simulink model "Combined"  (R2021b)
settings: Solver=FixedStepAuto  StartTime=0.0  StopTime=inf  FixedStep=0.001  RelTol=1e-3  EnableMultiTasking=on
undefined symbols (not defined in the file): D0, D1, D10, D11, D12, D13, D2, D3, D4, D5, D6, D7, D8, D9, PTA0, PTA1, PTA2, PTB23, PTB9, PTC16, PTC17, PTC2, PTC3, PTC4, PTD0, PTD1, PTD2, PTD3
libraries: simulink x25, frdmk64flib x15
(part 1 of 2)
settings Model: ExtModeTrigDuration=5  Creator=12268  LastModifiedBy=Aaron
settings SolverCC: AlgebraicLoopSolver=TrustRegion
settings OptimizationCC: EnhancedBackFolding=on  PassReuseOutputArgsAs=Individual arguments  ZeroExternalMemoryAtStartup=off  ZeroInternalMemoryAtStartup=off  MaxStackSize=64  OptimizeBlockOrder=speed  DifferentSizesBufferReuse=on  OptimizationCustomize=off  EfficientTunableParamExpr=on
settings DebuggingCC: ParameterTunabilityLossMsg=error  SFMachineParentedDataDiag=warning
settings HardwareCC: ProdBitPerPointer=32  ProdBitPerSizeT=32  ProdBitPerPtrDiffT=32  ProdLargestAtomicInteger=Long  ProdLargestAtomicFloat=Double  ProdWordSize=32  ProdHWDeviceType=ARM Compatible->ARM Cortex
settings SFSimCC: MATLABDynamicMemAlloc=off
settings RTWCC: Description=Embedded Coder  SystemTargetFile=ert.tlc  HardwareBoard=NXP FRDM-K64F  TLCOptions="-aInlineSetEventsForThisBaseRateFcn=TLC_FALSE -aSuppressMultiTaskScheduler=TLC_FALSE  -aRateBasedStepFcn=0"  TemplateMakefile=ert_default_tmf  Toolchain=GNU Tools for ARM Embedded Processors
settings CodeAppCC: ForceParamTrailComments=on  IgnoreCustomStorageClasses=off  OperatorAnnotations=on  SimulinkDataObjDesc=on  SFDataObjDesc=on  InsertBlockDesc=on

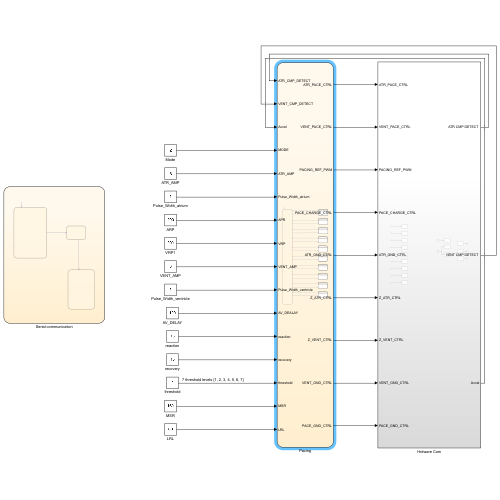
[thumbnail: Simulink's stored preview of the top-level diagram]
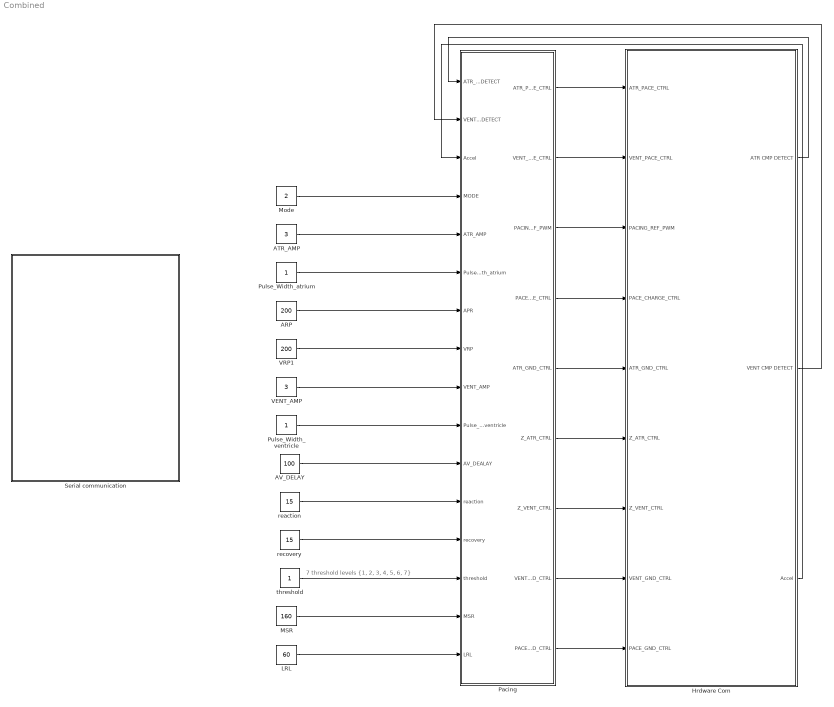
== system Combined ==
  note: 7 threshold levels {1, 2, 3, 4, 5, 6, 7}
  ARP : Constant  Value=200  OutDataTypeStr=uint16
  ATR_AMP : Constant  Value=3  OutDataTypeStr=double
  AV_DELAY : Constant  Value=100  OutDataTypeStr=uint16
  Hrdware Com : Subsystem
  LRL : Constant  Value=60
  MSR : Constant  Value=160
  Mode : Constant  Value=2  OutDataTypeStr=uint8
  Pacing : Stateflow chart  TreatAsAtomicUnit=on
      settings: PortSchema="{\"entries\":[{\"content\":{\"sides\":[{\"content\":{\"connectorIds\":[\"In1\",\"In2\",\"In3\",\"In4\",\"In5\",\"In6\",\"In8\",\"In9\",\"In16\",\"In10\",\"In11\",\"In12\",\"In13\",\"In14\",\"In15\",\"In7\"]},\"type\":\"ConnectorPlacement.EquallySpacedRectSide\",\"uuid\":\"b899f434-ac53-4776-90ad-1e47a9a70434\"},{\"content\":{\"connectorIds\":[\"Out1\",\"Out2\",\"Out3\",\"Out4\",\"Out5\",\"Out6\",\"Out7\",\"Out8\",\"Out9\"],\"side\":\"RIGHT\"},\"type\":\"ConnectorPlacement.EquallySpacedRectSide\",\"uuid\":\"a7a3dadf-3ead-4ae9-aa27-961636c111e5\"},{\"content\":{\"connectorIds\":[],\"side\":\"TOP\"},\"type\":\"ConnectorPlacement.EquallySpacedRectSide\",\"uuid\":\"97214a2f-6b07-43aa-affc-b9c6648cc812\"}]},\"type\":\"ConnectorPlacement.EquallySpacedConnector\",\"uuid\":\"1a78d035-42b2-4799-ac0c-6d5f965b7fff\"}],\"packageUris\":[\"http://schema.mathworks.com/mf0/Connector/R2020b\"],\"version\":\"1.0\"}"
  Pulse_Width_atrium : Constant  OutDataTypeStr=uint16
  Pulse_Width_ventricle : Constant  OutDataTypeStr=uint16
  Serial communication : Stateflow chart  TreatAsAtomicUnit=on
  VENT_AMP : Constant  Value=3  OutDataTypeStr=uint16
  VRP1 : Constant  Value=200  OutDataTypeStr=uint16
  reaction : Constant  Value=15  OutDataTypeStr=double
  recovery : Constant  Value=15  OutDataTypeStr=double
  threshold : Constant  OutDataTypeStr=single
  wires:
  Mode/1 -> Pacing/4(MODE)
  Pulse_Width_atrium/1 -> Pacing/6(Pulse_Width_atrium)
  ATR_AMP/1 -> Pacing/5(ATR_AMP)
  Pacing/1(ATR_PACE_CTRL) -> Hrdware Com/1(ATR_PACE_CTRL)
  Pacing/2(VENT_PACE_CTRL) -> Hrdware Com/2(VENT_PACE_CTRL)
  Pacing/3(PACING_REF_PWM) -> Hrdware Com/3(PACING_REF_PWM)
  Pacing/4(PACE_CHARGE_CTRL) -> Hrdware Com/4(PACE_CHARGE_CTRL)
  Pacing/5(ATR_GND_CTRL) -> Hrdware Com/5(ATR_GND_CTRL)
  Pacing/6(Z_ATR_CTRL) -> Hrdware Com/6("Z_ATR_CTRL ")
  Pacing/8(VENT_GND_CTRL) -> Hrdware Com/8(VENT_GND_CTRL)
  Pacing/9(PACE_GND_CTRL) -> Hrdware Com/9(PACE_GND_CTRL)
  Pacing/7(Z_VENT_CTRL) -> Hrdware Com/7("Z_VENT_CTRL ")
  ARP/1 -> Pacing/8(APR)
  Hrdware Com/1("ATR CMP DETECT ") -> Pacing/1(ATR_CMP_DETECT)
  Hrdware Com/2("VENT CMP DETECT ") -> Pacing/2(VENT_CMP_DETECT)
  VRP1/1 -> Pacing/9(VRP)
  Pulse_Width_ventricle/1 -> Pacing/10(Pulse_Width_ventricle)
  AV_DELAY/1 -> Pacing/11(AV_DEALAY)
  reaction/1 -> Pacing/12(reaction)
  threshold/1 -> Pacing/14(threshold)
  MSR/1 -> Pacing/15(MSR)
  LRL/1 -> Pacing/7(LRL)
  recovery/1 -> Pacing/13(recovery)
  Hrdware Com/3(Accel) -> Pacing/3(Accel)
  VENT_AMP/1 -> Pacing/16(VENT_AMP)

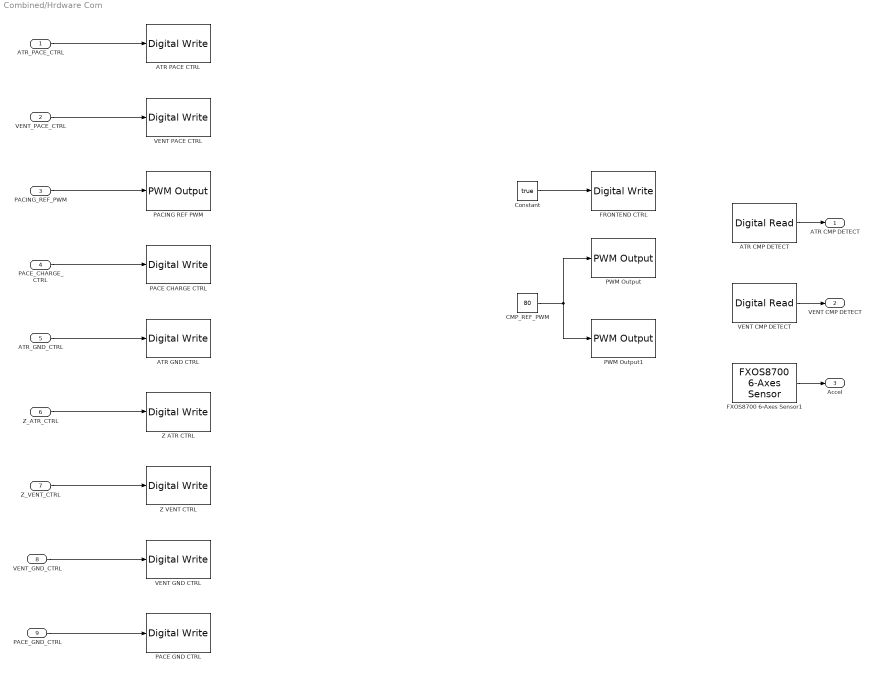
== system Combined/Hrdware Com ==
  ATR_PACE_CTRL : Inport
  VENT_PACE_CTRL : Inport  Port=2
  PACING_REF_PWM : Inport  Port=3
  PACE_CHARGE_CTRL : Inport  Port=4
  ATR_GND_CTRL : Inport  Port=5
  "Z_ATR_CTRL " : Inport  Port=6
  "Z_VENT_CTRL " : Inport  Port=7
  VENT_GND_CTRL : Inport  Port=8
  PACE_GND_CTRL : Inport  Port=9
  ATR CMP DETECT : frdmk64flib/Digital Read  Whichpin=PTC16 (D0)  SampleTime=-1
  "ATR GND CTRL " : frdmk64flib/Digital Write  Whichpin=PTD2 (D11)
  ATR PACE CTRL : frdmk64flib/Digital Write  Whichpin=PTA0 (D8)
  CMP_REF_PWM : Constant  Value=80  OutDataTypeStr=double
  Constant : Constant  Value=true  OutDataTypeStr=boolean
  FRONTEND CTRL : frdmk64flib/Digital Write  Whichpin=PTD1 (D13)
  FXOS8700 6-Axes Sensor1 : frdmk64flib/FXOS8700 6-Axes Sensor  Activesensor=Accelerometer only  ODR=800Hz  HybridODR=400Hz  Accelfullrange=-2g to +2g  SampleTime=-1
  PACE CHARGE CTRL : frdmk64flib/Digital Write  Whichpin=PTB9 (D2)
  PACE GND CTRL : frdmk64flib/Digital Write  Whichpin=PTD0 (D10)
  PACING REF PWM : frdmk64flib/PWM Output  Whichpin=PTA2 (D5)  InitialFrequency=2000  InitialDutyCycle=0
  PWM Output : frdmk64flib/PWM Output  Whichpin=PTC2 (D6)  InitialFrequency=2000  InitialDutyCycle=0
  PWM Output1 : frdmk64flib/PWM Output  Whichpin=PTA1 (D3)  InitialFrequency=2000  InitialDutyCycle=0
  VENT CMP DETECT : frdmk64flib/Digital Read  Whichpin=PTC17 (D1)  SampleTime=-1
  VENT GND CTRL : frdmk64flib/Digital Write  Whichpin=PTD3 (D12)
  VENT PACE CTRL : frdmk64flib/Digital Write  Whichpin=PTC4 (D9)
  "Z ATR CTRL " : frdmk64flib/Digital Write  Whichpin=PTB23 (D4)
  "Z VENT CTRL " : frdmk64flib/Digital Write  Whichpin=PTC3 (D7)
  "ATR CMP DETECT " : Outport  OutDataTypeStr=boolean  PortDimensions=1
  "VENT CMP DETECT " : Outport  Port=2  OutDataTypeStr=boolean  PortDimensions=1
  Accel : Outport  Port=3  OutDataTypeStr=boolean  PortDimensions=1
  wires:
  ATR_PACE_CTRL/1 -> ATR PACE CTRL/1
  VENT_PACE_CTRL/1 -> VENT PACE CTRL/1
  PACING_REF_PWM/1 -> PACING REF PWM/1
  PACE_CHARGE_CTRL/1 -> PACE CHARGE CTRL/1
  ATR_GND_CTRL/1 -> "ATR GND CTRL "/1
  "Z_ATR_CTRL "/1 -> "Z ATR CTRL "/1
  "Z_VENT_CTRL "/1 -> "Z VENT CTRL "/1
  VENT_GND_CTRL/1 -> VENT GND CTRL/1
  PACE_GND_CTRL/1 -> PACE GND CTRL/1
  Constant/1 -> FRONTEND CTRL/1
  ATR CMP DETECT/1 -> "ATR CMP DETECT "/1
  CMP_REF_PWM/1 -> PWM Output/1, PWM Output1/1
  VENT CMP DETECT/1 -> "VENT CMP DETECT "/1
  FXOS8700 6-Axes Sensor1/1 -> Accel/1

== system Combined/Pacing/AAI ==
  ATR_AMP : Inport
  Pulse_Width_atrium : Inport  Port=2
  LRL : Inport  Port=3
  APR : Inport  Port=4
  ATR_CMP_DETECT : Inport  Port=5
  Action Port : ActionPort
      settings: CopyFcn=Stateflow.SLINSF.SimulinkMan.removeBlockPreDeleteFcn  PreDeleteFcn=Stateflow.SLINSF.SimulinkMan.unsafePredeleteFcn
  "BPM to msec/B " : Subsystem
  Chart1 : Stateflow chart  TreatAsAtomicUnit=on
  ATR_PACE_CTRL : Outport
  VENT_PACE_CTRL : Outport  Port=2
  PACING_REF_PWM : Outport  Port=3
  PACE_CHARGE_CTRL : Outport  Port=4
  ATR_GND_CTRL : Outport  Port=5
  Z_ATR_CTRL : Outport  Port=6
  Z_VENT_CTRL : Outport  Port=7
  VENT_GND_CTRL : Outport  Port=8
  PACE_GND_CTRL : Outport  Port=9
  wires:
  Chart1/9(PACE_GND_CTRL) -> PACE_GND_CTRL/1
  Chart1/2(VENT_PACE_CTRL) -> VENT_PACE_CTRL/1
  Chart1/4(PACE_CHARGE_CTRL) -> PACE_CHARGE_CTRL/1
  Chart1/8(VENT_GND_CTRL) -> VENT_GND_CTRL/1
  Chart1/5(ATR_GND_CTRL) -> ATR_GND_CTRL/1
  Chart1/3(PACING_REF_PWM) -> PACING_REF_PWM/1
  Chart1/7(Z_VENT_CTRL) -> Z_VENT_CTRL/1
  Chart1/6(Z_ATR_CTRL) -> Z_ATR_CTRL/1
  Chart1/1(ATR_PACE_CTRL) -> ATR_PACE_CTRL/1
  ATR_AMP/1 -> Chart1/3(Amplitude)
  LRL/1 -> "BPM to msec/B "/1(LRL)
  Pulse_Width_atrium/1 -> Chart1/4(PULSE_WIDTH)
  APR/1 -> Chart1/2(ARP)
  "BPM to msec/B "/1(Out1) -> Chart1/5(LRL)
  ATR_CMP_DETECT/1 -> Chart1/1(SENSED)

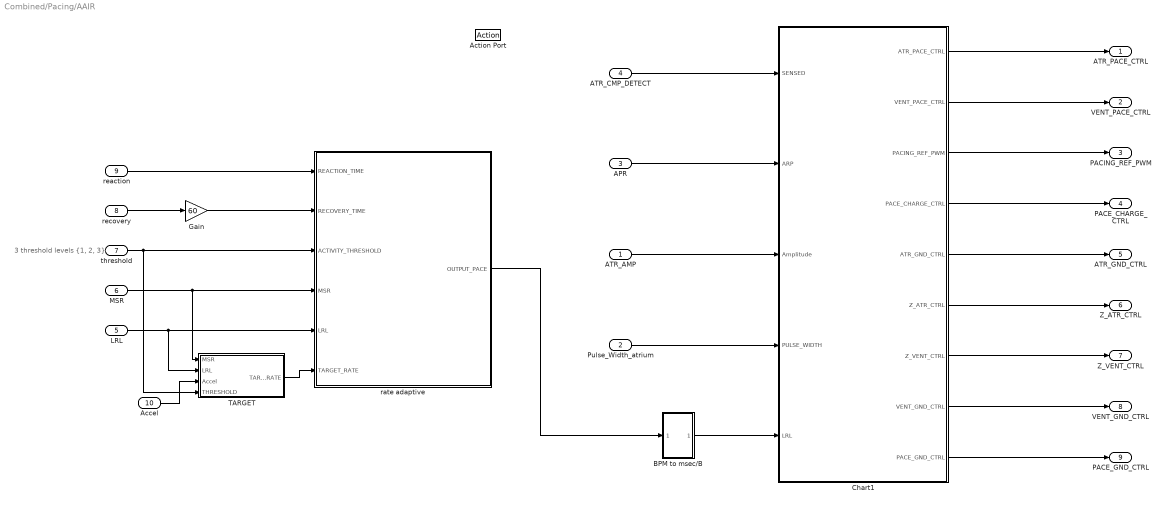
== system Combined/Pacing/AAIR ==
  note: 3 threshold levels {1, 2, 3}
  ATR_AMP : Inport
  Pulse_Width_atrium : Inport  Port=2
  APR : Inport  Port=3
  ATR_CMP_DETECT : Inport  Port=4
  LRL : Inport  Port=5
  MSR : Inport  Port=6
  threshold : Inport  Port=7
  recovery : Inport  Port=8
  reaction : Inport  Port=9
  Accel : Inport  Port=10
  Action Port : ActionPort
      settings: CopyFcn=Stateflow.SLINSF.SimulinkMan.removeBlockPreDeleteFcn  PreDeleteFcn=Stateflow.SLINSF.SimulinkMan.unsafePredeleteFcn
  "BPM to msec/B " : Subsystem
  Chart1 : Stateflow chart  TreatAsAtomicUnit=on
  Gain : Gain  Gain=60
  TARGET : Subsystem
  rate adaptive : Stateflow chart  TreatAsAtomicUnit=on
      settings: PortSchema="{\"entries\":[{\"content\":{\"sides\":[{\"content\":{\"connectorIds\":[\"In3\",\"In4\",\"In5\",\"In1\",\"In2\",\"In6\"]},\"type\":\"ConnectorPlacement.EquallySpacedRectSide\",\"uuid\":\"d3aa46b7-da68-4733-bd03-102d604fce17\"},{\"content\":{\"connectorIds\":[\"Out1\"],\"side\":\"RIGHT\"},\"type\":\"ConnectorPlacement.EquallySpacedRectSide\",\"uuid\":\"afbb636e-6b76-41fa-bb75-ca0d3f63044e\"},{\"content\":{\"connectorIds\":[],\"side\":\"TOP\"},\"type\":\"ConnectorPlacement.EquallySpacedRectSide\",\"uuid\":\"40571637-2e0f-45fd-89f0-6c332ecbd683\"}]},\"type\":\"ConnectorPlacement.EquallySpacedConnector\",\"uuid\":\"5e4e3dcb-fc0d-40cc-8fd4-4ca115cadd01\"}],\"packageUris\":[\"http://schema.mathworks.com/mf0/Connector/R2020b\"],\"version\":\"1.0\"}"
  ATR_PACE_CTRL : Outport
  VENT_PACE_CTRL : Outport  Port=2
  PACING_REF_PWM : Outport  Port=3
  PACE_CHARGE_CTRL : Outport  Port=4
  ATR_GND_CTRL : Outport  Port=5
  Z_ATR_CTRL : Outport  Port=6
  Z_VENT_CTRL : Outport  Port=7
  VENT_GND_CTRL : Outport  Port=8
  PACE_GND_CTRL : Outport  Port=9
  wires:
  recovery/1 -> Gain/1
  threshold/1 -> TARGET/4(THRESHOLD), rate adaptive/5(ACTIVITY_THRESHOLD)
  LRL/1 -> rate adaptive/2(LRL), TARGET/2(LRL)
  reaction/1 -> rate adaptive/3(REACTION_TIME)
  MSR/1 -> TARGET/1(MSR), rate adaptive/1(MSR)
  TARGET/1(TARGET_RATE) -> rate adaptive/6(TARGET_RATE)
  Gain/1 -> rate adaptive/4(RECOVERY_TIME)
  Chart1/9(PACE_GND_CTRL) -> PACE_GND_CTRL/1
  Chart1/6(Z_ATR_CTRL) -> Z_ATR_CTRL/1
  Chart1/7(Z_VENT_CTRL) -> Z_VENT_CTRL/1
  Chart1/8(VENT_GND_CTRL) -> VENT_GND_CTRL/1
  ATR_CMP_DETECT/1 -> Chart1/1(SENSED)
  Chart1/2(VENT_PACE_CTRL) -> VENT_PACE_CTRL/1
  Chart1/3(PACING_REF_PWM) -> PACING_REF_PWM/1
  Chart1/1(ATR_PACE_CTRL) -> ATR_PACE_CTRL/1
  APR/1 -> Chart1/2(ARP)
  Chart1/5(ATR_GND_CTRL) -> ATR_GND_CTRL/1
  Pulse_Width_atrium/1 -> Chart1/4(PULSE_WIDTH)
  Chart1/4(PACE_CHARGE_CTRL) -> PACE_CHARGE_CTRL/1
  "BPM to msec/B "/1(Out1) -> Chart1/5(LRL)
  rate adaptive/1(OUTPUT_PACE) -> "BPM to msec/B "/1(LRL)
  ATR_AMP/1 -> Chart1/3(Amplitude)
  Accel/1 -> TARGET/3(Accel)

== system Combined/Pacing/AOO ==
  ATR_AMP : Inport
  Pulse_Width_atrium : Inport  Port=2
  LRL : Inport  Port=3
  Action Port : ActionPort
      settings: CopyFcn=Stateflow.SLINSF.SimulinkMan.removeBlockPreDeleteFcn  PreDeleteFcn=Stateflow.SLINSF.SimulinkMan.unsafePredeleteFcn
  "BPM to msec/B " : Subsystem
  Chart : Stateflow chart  TreatAsAtomicUnit=on
  ATR_PACE_CTRL : Outport
  VENT_PACE_CTRL : Outport  Port=2
  PACING_REF_PWM : Outport  Port=3
  PACE_CHARGE_CTRL : Outport  Port=4
  ATR_GND_CTRL : Outport  Port=5
  Z_ATR_CTRL : Outport  Port=6
  Z_VENT_CTRL : Outport  Port=7
  VENT_GND_CTRL : Outport  Port=8
  PACE_GND_CTRL : Outport  Port=9
  wires:
  Chart/6(Z_ATR_CTRL) -> Z_ATR_CTRL/1
  Chart/8(VENT_GND_CTRL) -> VENT_GND_CTRL/1
  Chart/4(PACE_CHARGE_CTRL) -> PACE_CHARGE_CTRL/1
  Chart/9(PACE_GND_CTRL) -> PACE_GND_CTRL/1
  Chart/3(PACING_REF_PWM) -> PACING_REF_PWM/1
  Chart/1(ATR_PACE_CTRL) -> ATR_PACE_CTRL/1
  Chart/7(Z_VENT_CTRL) -> Z_VENT_CTRL/1
  Chart/5(ATR_GND_CTRL) -> ATR_GND_CTRL/1
  Chart/2(VENT_PACE_CTRL) -> VENT_PACE_CTRL/1
  ATR_AMP/1 -> Chart/1(Amplitude)
  Pulse_Width_atrium/1 -> Chart/2(PULSE_WIDTH)
  "BPM to msec/B "/1(Out1) -> Chart/3(LRL)
  LRL/1 -> "BPM to msec/B "/1(LRL)

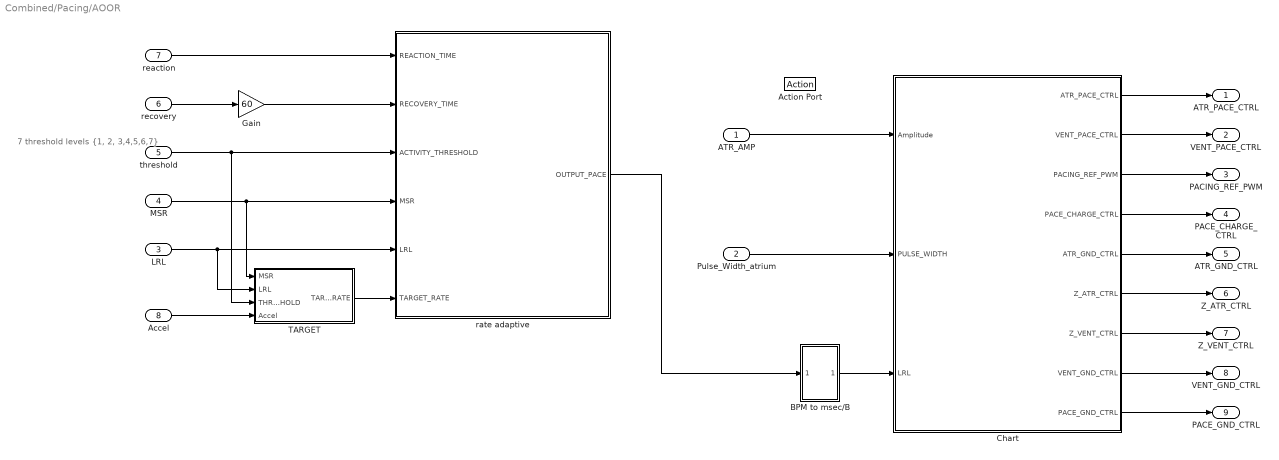
== system Combined/Pacing/AOOR ==
  note: 7 threshold levels {1, 2, 3,4,5,6,7}
  ATR_AMP : Inport
  Pulse_Width_atrium : Inport  Port=2
  LRL : Inport  Port=3
  MSR : Inport  Port=4
  threshold : Inport  Port=5
  recovery : Inport  Port=6
  reaction : Inport  Port=7
  Accel : Inport  Port=8
  Action Port : ActionPort
      settings: CopyFcn=Stateflow.SLINSF.SimulinkMan.removeBlockPreDeleteFcn  PreDeleteFcn=Stateflow.SLINSF.SimulinkMan.unsafePredeleteFcn
  "BPM to msec/B " : Subsystem
  Chart : Stateflow chart  TreatAsAtomicUnit=on
  Gain : Gain  Gain=60
  TARGET : Subsystem
  rate adaptive : Stateflow chart  TreatAsAtomicUnit=on
      settings: PortSchema="{\"entries\":[{\"content\":{\"sides\":[{\"content\":{\"connectorIds\":[\"In3\",\"In4\",\"In5\",\"In1\",\"In2\",\"In6\"]},\"type\":\"ConnectorPlacement.EquallySpacedRectSide\",\"uuid\":\"d3aa46b7-da68-4733-bd03-102d604fce17\"},{\"content\":{\"connectorIds\":[\"Out1\"],\"side\":\"RIGHT\"},\"type\":\"ConnectorPlacement.EquallySpacedRectSide\",\"uuid\":\"afbb636e-6b76-41fa-bb75-ca0d3f63044e\"},{\"content\":{\"connectorIds\":[],\"side\":\"TOP\"},\"type\":\"ConnectorPlacement.EquallySpacedRectSide\",\"uuid\":\"40571637-2e0f-45fd-89f0-6c332ecbd683\"}]},\"type\":\"ConnectorPlacement.EquallySpacedConnector\",\"uuid\":\"5e4e3dcb-fc0d-40cc-8fd4-4ca115cadd01\"}],\"packageUris\":[\"http://schema.mathworks.com/mf0/Connector/R2020b\"],\"version\":\"1.0\"}"
  ATR_PACE_CTRL : Outport
  VENT_PACE_CTRL : Outport  Port=2
  PACING_REF_PWM : Outport  Port=3
  PACE_CHARGE_CTRL : Outport  Port=4
  ATR_GND_CTRL : Outport  Port=5
  Z_ATR_CTRL : Outport  Port=6
  Z_VENT_CTRL : Outport  Port=7
  VENT_GND_CTRL : Outport  Port=8
  PACE_GND_CTRL : Outport  Port=9
  wires:
  Chart/9(PACE_GND_CTRL) -> PACE_GND_CTRL/1
  Chart/2(VENT_PACE_CTRL) -> VENT_PACE_CTRL/1
  Chart/4(PACE_CHARGE_CTRL) -> PACE_CHARGE_CTRL/1
  Chart/8(VENT_GND_CTRL) -> VENT_GND_CTRL/1
  Chart/5(ATR_GND_CTRL) -> ATR_GND_CTRL/1
  Chart/3(PACING_REF_PWM) -> PACING_REF_PWM/1
  Chart/7(Z_VENT_CTRL) -> Z_VENT_CTRL/1
  Chart/6(Z_ATR_CTRL) -> Z_ATR_CTRL/1
  Chart/1(ATR_PACE_CTRL) -> ATR_PACE_CTRL/1
  ATR_AMP/1 -> Chart/1(Amplitude)
  Pulse_Width_atrium/1 -> Chart/2(PULSE_WIDTH)
  Gain/1 -> rate adaptive/4(RECOVERY_TIME)
  "BPM to msec/B "/1(Out1) -> Chart/3(LRL)
  rate adaptive/1(OUTPUT_PACE) -> "BPM to msec/B "/1(In1)
  reaction/1 -> rate adaptive/3(REACTION_TIME)
  recovery/1 -> Gain/1
  threshold/1 -> TARGET/3(THRESHOLD), rate adaptive/5(ACTIVITY_THRESHOLD)
  MSR/1 -> TARGET/1(MSR), rate adaptive/1(MSR)
  TARGET/1(TARGET_RATE) -> rate adaptive/6(TARGET_RATE)
  LRL/1 -> rate adaptive/2(LRL), TARGET/2(LRL)
  Accel/1 -> TARGET/4(Accel)

== system Combined/Pacing/DOO ==
  VENT_AMP : Inport
  Pulse_Width_atrium : Inport  Port=2
  LRL : Inport  Port=3
  Pulse_Width_ventricle : Inport  Port=4
  AV_DEALAY : Inport  Port=5
  ATR_AMP : Inport  Port=6
  Action Port : ActionPort
      settings: CopyFcn=Stateflow.SLINSF.SimulinkMan.removeBlockPreDeleteFcn  PreDeleteFcn=Stateflow.SLINSF.SimulinkMan.unsafePredeleteFcn
  "BPM to msec/B " : Subsystem
  Chart : Stateflow chart  TreatAsAtomicUnit=on
      settings: PortSchema="{\"entries\":[{\"content\":{\"sides\":[{\"content\":{\"connectorIds\":[\"In1\",\"In6\",\"In5\",\"In2\",\"In3\",\"In4\"]},\"type\":\"ConnectorPlacement.EquallySpacedRectSide\",\"uuid\":\"72970874-2a7f-4f54-9c96-49c3612305c0\"},{\"content\":{\"connectorIds\":[\"Out1\",\"Out2\",\"Out3\",\"Out4\",\"Out5\",\"Out6\",\"Out7\",\"Out8\",\"Out9\"],\"side\":\"RIGHT\"},\"type\":\"ConnectorPlacement.EquallySpacedRectSide\",\"uuid\":\"785d6d73-c00d-4bb6-bac4-9062a7713100\"},{\"content\":{\"connectorIds\":[],\"side\":\"TOP\"},\"type\":\"ConnectorPlacement.EquallySpacedRectSide\",\"uuid\":\"f7c58201-4adc-48cf-bf7a-118db90373b1\"}]},\"type\":\"ConnectorPlacement.EquallySpacedConnector\",\"uuid\":\"33960bc4-ecd9-4e8c-b37b-5f7b6e376475\"}],\"packageUris\":[\"http://schema.mathworks.com/mf0/Connector/R2020b\"],\"version\":\"1.0\"}"
  ATR_PACE_CTRL : Outport
  VENT_PACE_CTRL : Outport  Port=2
  PACING_REF_PWM : Outport  Port=3
  PACE_CHARGE_CTRL : Outport  Port=4
  ATR_GND_CTRL : Outport  Port=5
  Z_ATR_CTRL : Outport  Port=6
  Z_VENT_CTRL : Outport  Port=7
  VENT_GND_CTRL : Outport  Port=8
  PACE_GND_CTRL : Outport  Port=9
  wires:
  Chart/9(PACE_GND_CTRL) -> PACE_GND_CTRL/1
  AV_DEALAY/1 -> Chart/5(AV_DELAY)
  "BPM to msec/B "/1(Out1) -> Chart/4(INTERVAL)
  Chart/3(PACING_REF_PWM) -> PACING_REF_PWM/1
  Pulse_Width_atrium/1 -> Chart/3(ATR_PULSE_WIDTH)
  Chart/8(VENT_GND_CTRL) -> VENT_GND_CTRL/1
  VENT_AMP/1 -> Chart/1(V_Amplitude)
  LRL/1 -> "BPM to msec/B "/1(In1)
  Chart/5(ATR_GND_CTRL) -> ATR_GND_CTRL/1
  Chart/4(PACE_CHARGE_CTRL) -> PACE_CHARGE_CTRL/1
  Chart/2(VENT_PACE_CTRL) -> VENT_PACE_CTRL/1
  Pulse_Width_ventricle/1 -> Chart/2(VENT_PULSE_WIDTH)
  Chart/1(ATR_PACE_CTRL) -> ATR_PACE_CTRL/1
  Chart/6(Z_ATR_CTRL) -> Z_ATR_CTRL/1
  Chart/7(Z_VENT_CTRL) -> Z_VENT_CTRL/1
  ATR_AMP/1 -> Chart/6(A_Amplitude)

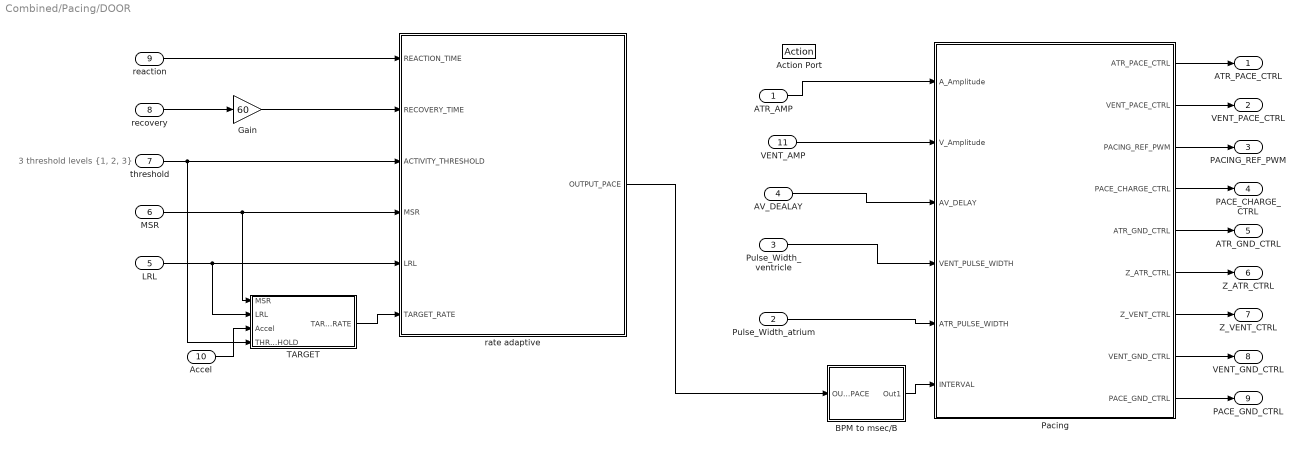
== system Combined/Pacing/DOOR ==
  note: 3 threshold levels {1, 2, 3}
  ATR_AMP : Inport
  Pulse_Width_atrium : Inport  Port=2
  Pulse_Width_ventricle : Inport  Port=3
  AV_DEALAY : Inport  Port=4
  LRL : Inport  Port=5
  MSR : Inport  Port=6
  threshold : Inport  Port=7
  recovery : Inport  Port=8
  reaction : Inport  Port=9
  Accel : Inport  Port=10
  VENT_AMP : Inport  Port=11
  Action Port : ActionPort
      settings: CopyFcn=Stateflow.SLINSF.SimulinkMan.removeBlockPreDeleteFcn  PreDeleteFcn=Stateflow.SLINSF.SimulinkMan.unsafePredeleteFcn
  "BPM to msec/B " : Subsystem
  Gain : Gain  Gain=60
  Pacing : Stateflow chart  TreatAsAtomicUnit=on
      settings: PortSchema="{\"entries\":[{\"content\":{\"sides\":[{\"content\":{\"connectorIds\":[\"In1\",\"In6\",\"In5\",\"In2\",\"In3\",\"In4\"]},\"type\":\"ConnectorPlacement.EquallySpacedRectSide\",\"uuid\":\"72970874-2a7f-4f54-9c96-49c3612305c0\"},{\"content\":{\"connectorIds\":[\"Out1\",\"Out2\",\"Out3\",\"Out4\",\"Out5\",\"Out6\",\"Out7\",\"Out8\",\"Out9\"],\"side\":\"RIGHT\"},\"type\":\"ConnectorPlacement.EquallySpacedRectSide\",\"uuid\":\"785d6d73-c00d-4bb6-bac4-9062a7713100\"},{\"content\":{\"connectorIds\":[],\"side\":\"TOP\"},\"type\":\"ConnectorPlacement.EquallySpacedRectSide\",\"uuid\":\"f7c58201-4adc-48cf-bf7a-118db90373b1\"}]},\"type\":\"ConnectorPlacement.EquallySpacedConnector\",\"uuid\":\"33960bc4-ecd9-4e8c-b37b-5f7b6e376475\"}],\"packageUris\":[\"http://schema.mathworks.com/mf0/Connector/R2020b\"],\"version\":\"1.0\"}"
  TARGET : Subsystem
  rate adaptive : Stateflow chart  TreatAsAtomicUnit=on
      settings: PortSchema="{\"entries\":[{\"content\":{\"sides\":[{\"content\":{\"connectorIds\":[\"In3\",\"In4\",\"In5\",\"In1\",\"In2\",\"In6\"]},\"type\":\"ConnectorPlacement.EquallySpacedRectSide\",\"uuid\":\"d3aa46b7-da68-4733-bd03-102d604fce17\"},{\"content\":{\"connectorIds\":[\"Out1\"],\"side\":\"RIGHT\"},\"type\":\"ConnectorPlacement.EquallySpacedRectSide\",\"uuid\":\"afbb636e-6b76-41fa-bb75-ca0d3f63044e\"},{\"content\":{\"connectorIds\":[],\"side\":\"TOP\"},\"type\":\"ConnectorPlacement.EquallySpacedRectSide\",\"uuid\":\"40571637-2e0f-45fd-89f0-6c332ecbd683\"}]},\"type\":\"ConnectorPlacement.EquallySpacedConnector\",\"uuid\":\"5e4e3dcb-fc0d-40cc-8fd4-4ca115cadd01\"}],\"packageUris\":[\"http://schema.mathworks.com/mf0/Connector/R2020b\"],\"version\":\"1.0\"}"
  ATR_PACE_CTRL : Outport
  VENT_PACE_CTRL : Outport  Port=2
  PACING_REF_PWM : Outport  Port=3
  PACE_CHARGE_CTRL : Outport  Port=4
  ATR_GND_CTRL : Outport  Port=5
  Z_ATR_CTRL : Outport  Port=6
  Z_VENT_CTRL : Outport  Port=7
  VENT_GND_CTRL : Outport  Port=8
  PACE_GND_CTRL : Outport  Port=9
  wires:
  Pulse_Width_atrium/1 -> Pacing/3(ATR_PULSE_WIDTH)
  Pacing/6(Z_ATR_CTRL) -> Z_ATR_CTRL/1
  Pacing/5(ATR_GND_CTRL) -> ATR_GND_CTRL/1
  rate adaptive/1(OUTPUT_PACE) -> "BPM to msec/B "/1(OUTPUT_PACE)
  Pacing/7(Z_VENT_CTRL) -> Z_VENT_CTRL/1
  AV_DEALAY/1 -> Pacing/5(AV_DELAY)
  "BPM to msec/B "/1(Out1) -> Pacing/4(INTERVAL)
  ATR_AMP/1 -> Pacing/1(A_Amplitude)
  Pacing/9(PACE_GND_CTRL) -> PACE_GND_CTRL/1
  Pacing/3(PACING_REF_PWM) -> PACING_REF_PWM/1
  Pacing/8(VENT_GND_CTRL) -> VENT_GND_CTRL/1
  Pacing/1(ATR_PACE_CTRL) -> ATR_PACE_CTRL/1
  Pacing/4(PACE_CHARGE_CTRL) -> PACE_CHARGE_CTRL/1
  Pulse_Width_ventricle/1 -> Pacing/2(VENT_PULSE_WIDTH)
  Pacing/2(VENT_PACE_CTRL) -> VENT_PACE_CTRL/1
  LRL/1 -> rate adaptive/2(LRL), TARGET/2(LRL)
  threshold/1 -> TARGET/4(THRESHOLD), rate adaptive/5(ACTIVITY_THRESHOLD)
  recovery/1 -> Gain/1
  MSR/1 -> TARGET/1(MSR), rate adaptive/1(MSR)
  reaction/1 -> rate adaptive/3(REACTION_TIME)
  Gain/1 -> rate adaptive/4(RECOVERY_TIME)
  TARGET/1(TARGET_RATE) -> rate adaptive/6(TARGET_RATE)
  Accel/1 -> TARGET/3(Accel)
  VENT_AMP/1 -> Pacing/6(V_Amplitude)

== system Combined/Pacing/VOO ==
  VENT_AMP : Inport
  Pulse_Width_ventricle : Inport  Port=2
  LRL : Inport  Port=3
  Action Port : ActionPort
      settings: CopyFcn=Stateflow.SLINSF.SimulinkMan.removeBlockPreDeleteFcn  PreDeleteFcn=Stateflow.SLINSF.SimulinkMan.unsafePredeleteFcn
  "BPM to msec/B " : Subsystem
  Chart : Stateflow chart  TreatAsAtomicUnit=on
  ATR_PACE_CTRL : Outport
  VENT_PACE_CTRL : Outport  Port=2
  PACING_REF_PWM : Outport  Port=3
  PACE_CHARGE_CTRL : Outport  Port=4
  ATR_GND_CTRL : Outport  Port=5
  Z_ATR_CTRL : Outport  Port=6
  Z_VENT_CTRL : Outport  Port=7
  VENT_GND_CTRL : Outport  Port=8
  PACE_GND_CTRL : Outport  Port=9
  wires:
  Chart/9(PACE_GND_CTRL) -> PACE_GND_CTRL/1
  Chart/2(VENT_PACE_CTRL) -> VENT_PACE_CTRL/1
  Chart/4(PACE_CHARGE_CTRL) -> PACE_CHARGE_CTRL/1
  Chart/8(VENT_GND_CTRL) -> VENT_GND_CTRL/1
  Chart/5(ATR_GND_CTRL) -> ATR_GND_CTRL/1
  Chart/3(PACING_REF_PWM) -> PACING_REF_PWM/1
  Chart/7(Z_VENT_CTRL) -> Z_VENT_CTRL/1
  Chart/6(Z_ATR_CTRL) -> Z_ATR_CTRL/1
  Chart/1(ATR_PACE_CTRL) -> ATR_PACE_CTRL/1
  VENT_AMP/1 -> Chart/1(Amplitude)
  Pulse_Width_ventricle/1 -> Chart/2(PULSE_WIDTH)
  "BPM to msec/B "/1(Out1) -> Chart/3(LRL)
  LRL/1 -> "BPM to msec/B "/1(LRL)

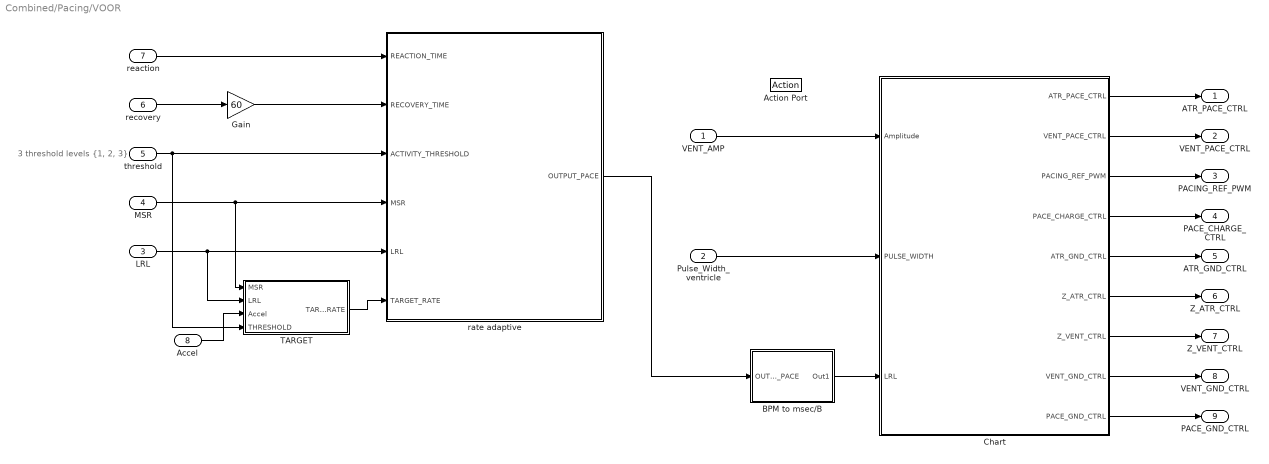
== system Combined/Pacing/VOOR ==
  note: 3 threshold levels {1, 2, 3}
  VENT_AMP : Inport
  Pulse_Width_ventricle : Inport  Port=2
  LRL : Inport  Port=3
  MSR : Inport  Port=4
  threshold : Inport  Port=5
  recovery : Inport  Port=6
  reaction : Inport  Port=7
  Accel : Inport  Port=8
  Action Port : ActionPort
      settings: CopyFcn=Stateflow.SLINSF.SimulinkMan.removeBlockPreDeleteFcn  PreDeleteFcn=Stateflow.SLINSF.SimulinkMan.unsafePredeleteFcn
  "BPM to msec/B " : Subsystem
  Chart : Stateflow chart  TreatAsAtomicUnit=on
  Gain : Gain  Gain=60
  TARGET : Subsystem
  rate adaptive : Stateflow chart  TreatAsAtomicUnit=on
      settings: PortSchema="{\"entries\":[{\"content\":{\"sides\":[{\"content\":{\"connectorIds\":[\"In3\",\"In4\",\"In5\",\"In1\",\"In2\",\"In6\"]},\"type\":\"ConnectorPlacement.EquallySpacedRectSide\",\"uuid\":\"d3aa46b7-da68-4733-bd03-102d604fce17\"},{\"content\":{\"connectorIds\":[\"Out1\"],\"side\":\"RIGHT\"},\"type\":\"ConnectorPlacement.EquallySpacedRectSide\",\"uuid\":\"afbb636e-6b76-41fa-bb75-ca0d3f63044e\"},{\"content\":{\"connectorIds\":[],\"side\":\"TOP\"},\"type\":\"ConnectorPlacement.EquallySpacedRectSide\",\"uuid\":\"40571637-2e0f-45fd-89f0-6c332ecbd683\"}]},\"type\":\"ConnectorPlacement.EquallySpacedConnector\",\"uuid\":\"5e4e3dcb-fc0d-40cc-8fd4-4ca115cadd01\"}],\"packageUris\":[\"http://schema.mathworks.com/mf0/Connector/R2020b\"],\"version\":\"1.0\"}"
  ATR_PACE_CTRL : Outport
  VENT_PACE_CTRL : Outport  Port=2
  PACING_REF_PWM : Outport  Port=3
  PACE_CHARGE_CTRL : Outport  Port=4
  ATR_GND_CTRL : Outport  Port=5
  Z_ATR_CTRL : Outport  Port=6
  Z_VENT_CTRL : Outport  Port=7
  VENT_GND_CTRL : Outport  Port=8
  PACE_GND_CTRL : Outport  Port=9
  wires:
  Chart/9(PACE_GND_CTRL) -> PACE_GND_CTRL/1
  Chart/2(VENT_PACE_CTRL) -> VENT_PACE_CTRL/1
  Chart/4(PACE_CHARGE_CTRL) -> PACE_CHARGE_CTRL/1
  Chart/8(VENT_GND_CTRL) -> VENT_GND_CTRL/1
  Chart/5(ATR_GND_CTRL) -> ATR_GND_CTRL/1
  Chart/3(PACING_REF_PWM) -> PACING_REF_PWM/1
  Chart/7(Z_VENT_CTRL) -> Z_VENT_CTRL/1
  Chart/6(Z_ATR_CTRL) -> Z_ATR_CTRL/1
  Chart/1(ATR_PACE_CTRL) -> ATR_PACE_CTRL/1
  recovery/1 -> Gain/1
  Gain/1 -> rate adaptive/4(RECOVERY_TIME)
  reaction/1 -> rate adaptive/3(REACTION_TIME)
  LRL/1 -> rate adaptive/2(LRL), TARGET/2(LRL)
  MSR/1 -> TARGET/1(MSR), rate adaptive/1(MSR)
  Pulse_Width_ventricle/1 -> Chart/2(PULSE_WIDTH)
  threshold/1 -> TARGET/4(THRESHOLD), rate adaptive/5(ACTIVITY_THRESHOLD)
  rate adaptive/1(OUTPUT_PACE) -> "BPM to msec/B "/1(OUTPUT_PACE)
  "BPM to msec/B "/1(Out1) -> Chart/3(LRL)
  VENT_AMP/1 -> Chart/1(Amplitude)
  TARGET/1(TARGET_RATE) -> rate adaptive/6(TARGET_RATE)
  Accel/1 -> TARGET/3(Accel)

== system Combined/Pacing/VVI ==
  VENT_AMP : Inport
  Pulse_Width_ventricle : Inport  Port=2
  LRL : Inport  Port=3
  VRP : Inport  Port=4
  VENT_CMP_DETECT : Inport  Port=5
  Action Port : ActionPort
      settings: CopyFcn=Stateflow.SLINSF.SimulinkMan.removeBlockPreDeleteFcn  PreDeleteFcn=Stateflow.SLINSF.SimulinkMan.unsafePredeleteFcn
  "BPM to msec/B " : Subsystem
  Chart : Stateflow chart  TreatAsAtomicUnit=on
  ATR_PACE_CTRL : Outport
  VENT_PACE_CTRL : Outport  Port=2
  PACING_REF_PWM : Outport  Port=3
  PACE_CHARGE_CTRL : Outport  Port=4
  ATR_GND_CTRL : Outport  Port=5
  Z_ATR_CTRL : Outport  Port=6
  Z_VENT_CTRL : Outport  Port=7
  VENT_GND_CTRL : Outport  Port=8
  PACE_GND_CTRL : Outport  Port=9
  wires:
  Chart/9(PACE_GND_CTRL) -> PACE_GND_CTRL/1
  Chart/6(Z_ATR_CTRL) -> Z_ATR_CTRL/1
  Chart/7(Z_VENT_CTRL) -> Z_VENT_CTRL/1
  Chart/8(VENT_GND_CTRL) -> VENT_GND_CTRL/1
  VENT_CMP_DETECT/1 -> Chart/1(SENSED)
  Chart/2(VENT_PACE_CTRL) -> VENT_PACE_CTRL/1
  Chart/3(PACING_REF_PWM) -> PACING_REF_PWM/1
  Chart/1(ATR_PACE_CTRL) -> ATR_PACE_CTRL/1
  VRP/1 -> Chart/2(VRP)
  Chart/5(ATR_GND_CTRL) -> ATR_GND_CTRL/1
  Pulse_Width_ventricle/1 -> Chart/4(PULSE_WIDTH)
  Chart/4(PACE_CHARGE_CTRL) -> PACE_CHARGE_CTRL/1
  "BPM to msec/B "/1(Out1) -> Chart/5(LRL)
  LRL/1 -> "BPM to msec/B "/1(LRL)
  VENT_AMP/1 -> Chart/3(Amplitude)

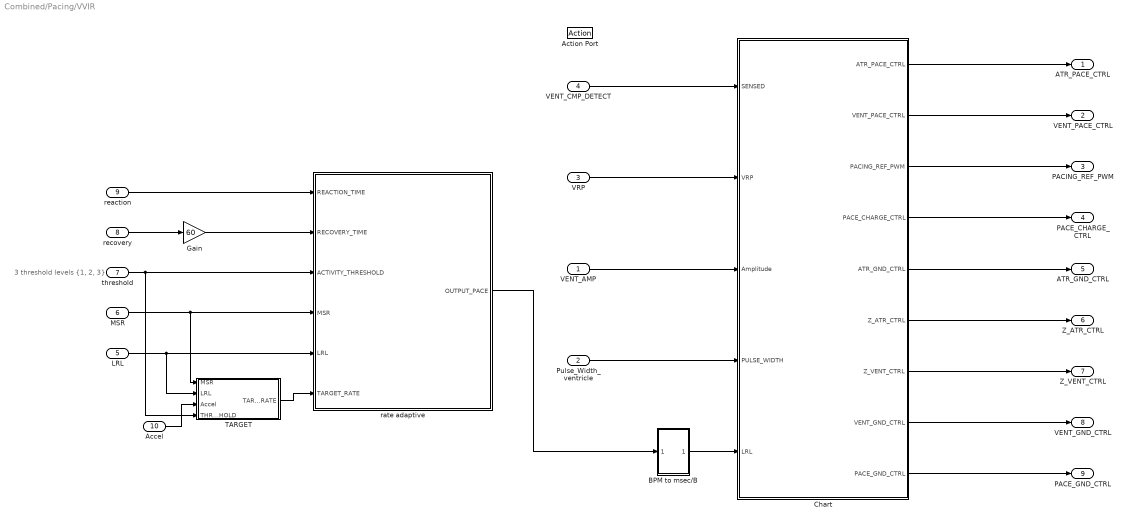
== system Combined/Pacing/VVIR ==
  note: 3 threshold levels {1, 2, 3}
  VENT_AMP : Inport
  Pulse_Width_ventricle : Inport  Port=2
  VRP : Inport  Port=3
  VENT_CMP_DETECT : Inport  Port=4
  LRL : Inport  Port=5
  MSR : Inport  Port=6
  threshold : Inport  Port=7
  recovery : Inport  Port=8
  reaction : Inport  Port=9
  Accel : Inport  Port=10
  Action Port : ActionPort
      settings: CopyFcn=Stateflow.SLINSF.SimulinkMan.removeBlockPreDeleteFcn  PreDeleteFcn=Stateflow.SLINSF.SimulinkMan.unsafePredeleteFcn
  "BPM to msec/B " : Subsystem
  Chart : Stateflow chart  TreatAsAtomicUnit=on
  Gain : Gain  Gain=60
  TARGET : Subsystem
  rate adaptive : Stateflow chart  TreatAsAtomicUnit=on
      settings: PortSchema="{\"entries\":[{\"content\":{\"sides\":[{\"content\":{\"connectorIds\":[\"In3\",\"In4\",\"In5\",\"In1\",\"In2\",\"In6\"]},\"type\":\"ConnectorPlacement.EquallySpacedRectSide\",\"uuid\":\"d3aa46b7-da68-4733-bd03-102d604fce17\"},{\"content\":{\"connectorIds\":[\"Out1\"],\"side\":\"RIGHT\"},\"type\":\"ConnectorPlacement.EquallySpacedRectSide\",\"uuid\":\"afbb636e-6b76-41fa-bb75-ca0d3f63044e\"},{\"content\":{\"connectorIds\":[],\"side\":\"TOP\"},\"type\":\"ConnectorPlacement.EquallySpacedRectSide\",\"uuid\":\"40571637-2e0f-45fd-89f0-6c332ecbd683\"}]},\"type\":\"ConnectorPlacement.EquallySpacedConnector\",\"uuid\":\"5e4e3dcb-fc0d-40cc-8fd4-4ca115cadd01\"}],\"packageUris\":[\"http://schema.mathworks.com/mf0/Connector/R2020b\"],\"version\":\"1.0\"}"
  ATR_PACE_CTRL : Outport
  VENT_PACE_CTRL : Outport  Port=2
  PACING_REF_PWM : Outport  Port=3
  PACE_CHARGE_CTRL : Outport  Port=4
  ATR_GND_CTRL : Outport  Port=5
  Z_ATR_CTRL : Outport  Port=6
  Z_VENT_CTRL : Outport  Port=7
  VENT_GND_CTRL : Outport  Port=8
  PACE_GND_CTRL : Outport  Port=9
  wires:
  VRP/1 -> Chart/2(VRP)
  VENT_CMP_DETECT/1 -> Chart/1(SENSED)
  "BPM to msec/B "/1(Out1) -> Chart/5(LRL)
  Pulse_Width_ventricle/1 -> Chart/4(PULSE_WIDTH)
  Chart/6(Z_ATR_CTRL) -> Z_ATR_CTRL/1
  Chart/8(VENT_GND_CTRL) -> VENT_GND_CTRL/1
  Chart/5(ATR_GND_CTRL) -> ATR_GND_CTRL/1
  Chart/2(VENT_PACE_CTRL) -> VENT_PACE_CTRL/1
  Chart/4(PACE_CHARGE_CTRL) -> PACE_CHARGE_CTRL/1
  Chart/3(PACING_REF_PWM) -> PACING_REF_PWM/1
  VENT_AMP/1 -> Chart/3(Amplitude)
  Chart/9(PACE_GND_CTRL) -> PACE_GND_CTRL/1
  Chart/1(ATR_PACE_CTRL) -> ATR_PACE_CTRL/1
  Chart/7(Z_VENT_CTRL) -> Z_VENT_CTRL/1
  MSR/1 -> TARGET/1(MSR), rate adaptive/1(MSR)
  rate adaptive/1(OUTPUT_PACE) -> "BPM to msec/B "/1(LRL)
  recovery/1 -> Gain/1
  threshold/1 -> TARGET/4(THRESHOLD), rate adaptive/5(ACTIVITY_THRESHOLD)
  LRL/1 -> rate adaptive/2(LRL), TARGET/2(LRL)
  TARGET/1(TARGET_RATE) -> rate adaptive/6(TARGET_RATE)
  Gain/1 -> rate adaptive/4(RECOVERY_TIME)
  reaction/1 -> rate adaptive/3(REACTION_TIME)
  Accel/1 -> TARGET/3(Accel)

== system Combined/Pacing/AAI/BPM to msec//B  ==
  LRL : Inport
  1 min(msec) : Constant  Value=60000  OutDataTypeStr=double
  "BPM to msec/B " : Product  Inputs=*/  OutDataTypeStr=uint16  RndMeth=Nearest
  Out1 : Outport
  wires:
  1 min(msec)/1 -> "BPM to msec/B "/1
  "BPM to msec/B "/1 -> Out1/1
  LRL/1 -> "BPM to msec/B "/2

== system Combined/Pacing/AAIR/BPM to msec//B  ==
  LRL : Inport
  1 min(msec) : Constant  Value=60000  OutDataTypeStr=double
  "BPM to msec/B " : Product  Inputs=*/  OutDataTypeStr=uint16  RndMeth=Nearest
  Out1 : Outport
  wires:
  1 min(msec)/1 -> "BPM to msec/B "/1
  "BPM to msec/B "/1 -> Out1/1
  LRL/1 -> "BPM to msec/B "/2

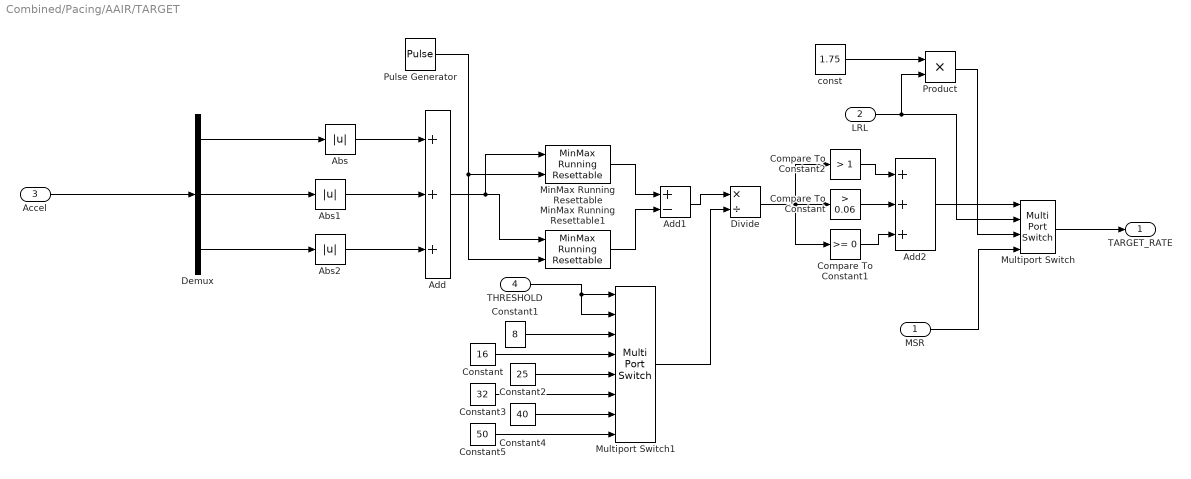
== system Combined/Pacing/AAIR/TARGET ==
  MSR : Inport
  LRL : Inport  Port=2
  Accel : Inport  Port=3
  THRESHOLD : Inport  Port=4
  Abs : Abs
  Abs1 : Abs
  Abs2 : Abs
  Add : Sum  Inputs=+++
  Add1 : Sum  Inputs=+-
  Add2 : Sum  Inputs=+++
  Compare To Constant : simulink/Logic and Bit Operations/Compare To Constant  relop=>  const=0.06  OutDataTypeStr=uint8
  Compare To Constant1 : simulink/Logic and Bit Operations/Compare To Constant  relop=>=  const=0  OutDataTypeStr=uint8
  Compare To Constant2 : simulink/Logic and Bit Operations/Compare To Constant  relop=>  const=1  OutDataTypeStr=uint8
  Constant : Constant  Value=16  OutDataTypeStr=single
  Constant1 : Constant  Value=8  OutDataTypeStr=single
  Constant2 : Constant  Value=25  OutDataTypeStr=single
  Constant3 : Constant  Value=32  OutDataTypeStr=single
  Constant4 : Constant  Value=40  OutDataTypeStr=single
  Constant5 : Constant  Value=50  OutDataTypeStr=single
  Demux : Demux  Outputs=3
  Divide : Product  Inputs=*/
  MinMax Running Resettable : simulink/Math Operations/MinMax Running Resettable  Function=max  vinit=1
  MinMax Running Resettable1 : simulink/Math Operations/MinMax Running Resettable  Function=min  vinit=1
  Multiport Switch : MultiPortSwitch  OutDataTypeStr=double
  Multiport Switch1 : MultiPortSwitch  Inputs=7
  Product : Product
  Pulse Generator : DiscretePulseGenerator  PulseType=Time based  PulseWidth=2.5
  const : Constant  Value=1.75
  TARGET_RATE : Outport
  wires:
  Compare To Constant/1 -> Add2/2
  Multiport Switch/1 -> TARGET_RATE/1
  Compare To Constant1/1 -> Add2/3
  Add2/1 -> Multiport Switch/1
  LRL/1 -> Product/2, Multiport Switch/2
  Product/1 -> Multiport Switch/3
  Abs2/1 -> Add/3
  Add/1 -> MinMax Running Resettable1/1, MinMax Running Resettable/1
  MinMax Running Resettable1/1 -> Add1/2
  Demux/2 -> Abs1/1
  Demux/3 -> Abs2/1
  Compare To Constant2/1 -> Add2/1
  MinMax Running Resettable/1 -> Add1/1
  Demux/1 -> Abs/1
  Pulse Generator/1 -> MinMax Running Resettable1/2, MinMax Running Resettable/2
  Abs/1 -> Add/1
  Abs1/1 -> Add/2
  Accel/1 -> Demux/1
  MSR/1 -> Multiport Switch/4
  const/1 -> Product/1
  Divide/1 -> Compare To Constant/1, Compare To Constant2/1, Compare To Constant1/1
  Add1/1 -> Divide/1
  Constant5/1 -> Multiport Switch1/8
  Constant3/1 -> Multiport Switch1/6
  Constant1/1 -> Multiport Switch1/3
  Constant2/1 -> Multiport Switch1/5
  Constant4/1 -> Multiport Switch1/7
  Constant/1 -> Multiport Switch1/4
  THRESHOLD/1 -> Multiport Switch1/2, Multiport Switch1/1
  Multiport Switch1/1 -> Divide/2

== system Combined/Pacing/AOO/BPM to msec//B  ==
  LRL : Inport
  1 min(msec) : Constant  Value=60000  OutDataTypeStr=double
  "BPM to msec/B " : Product  Inputs=*/  OutDataTypeStr=uint16  RndMeth=Nearest
  Out1 : Outport
  wires:
  1 min(msec)/1 -> "BPM to msec/B "/1
  "BPM to msec/B "/1 -> Out1/1
  LRL/1 -> "BPM to msec/B "/2

== system Combined/Pacing/AOOR/BPM to msec//B  ==
  In1 : Inport
  1 min(msec) : Constant  Value=60000  OutDataTypeStr=double
  "BPM to msec/B " : Product  Inputs=*/  OutDataTypeStr=uint16  RndMeth=Nearest
  Out1 : Outport
  wires:
  1 min(msec)/1 -> "BPM to msec/B "/1
  "BPM to msec/B "/1 -> Out1/1
  In1/1 -> "BPM to msec/B "/2

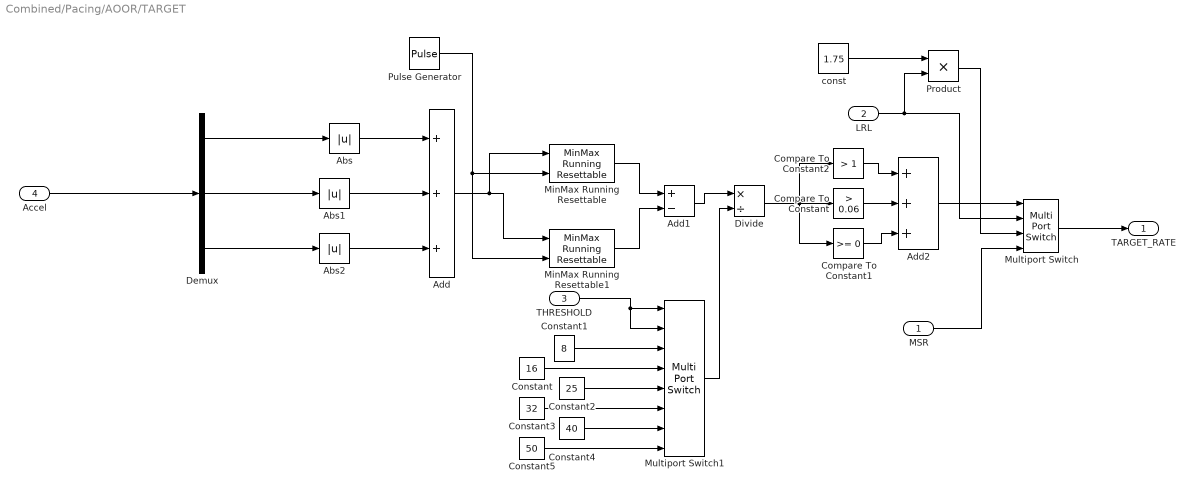
== system Combined/Pacing/AOOR/TARGET ==
  MSR : Inport
  LRL : Inport  Port=2
  THRESHOLD : Inport  Port=3
  Accel : Inport  Port=4
  Abs : Abs
  Abs1 : Abs
  Abs2 : Abs
  Add : Sum  Inputs=+++
  Add1 : Sum  Inputs=+-
  Add2 : Sum  Inputs=+++
  Compare To Constant : simulink/Logic and Bit Operations/Compare To Constant  relop=>  const=0.06  OutDataTypeStr=uint8
  Compare To Constant1 : simulink/Logic and Bit Operations/Compare To Constant  relop=>=  const=0  OutDataTypeStr=uint8
  Compare To Constant2 : simulink/Logic and Bit Operations/Compare To Constant  relop=>  const=1  OutDataTypeStr=uint8
  Constant : Constant  Value=16  OutDataTypeStr=single
  Constant1 : Constant  Value=8  OutDataTypeStr=single
  Constant2 : Constant  Value=25  OutDataTypeStr=single
  Constant3 : Constant  Value=32  OutDataTypeStr=single
  Constant4 : Constant  Value=40  OutDataTypeStr=single
  Constant5 : Constant  Value=50  OutDataTypeStr=single
  Demux : Demux  Outputs=3
  Divide : Product  Inputs=*/
  MinMax Running Resettable : simulink/Math Operations/MinMax Running Resettable  Function=max  vinit=1
  MinMax Running Resettable1 : simulink/Math Operations/MinMax Running Resettable  Function=min  vinit=1
  Multiport Switch : MultiPortSwitch  OutDataTypeStr=double
  Multiport Switch1 : MultiPortSwitch  Inputs=7
  Product : Product
  Pulse Generator : DiscretePulseGenerator  PulseType=Time based  PulseWidth=2.5
  const : Constant  Value=1.75
  TARGET_RATE : Outport
  wires:
  Compare To Constant/1 -> Add2/2
  Multiport Switch/1 -> TARGET_RATE/1
  Compare To Constant1/1 -> Add2/3
  Add2/1 -> Multiport Switch/1
  LRL/1 -> Product/2, Multiport Switch/2
  Product/1 -> Multiport Switch/3
  Abs2/1 -> Add/3
  Add/1 -> MinMax Running Resettable1/1, MinMax Running Resettable/1
  MinMax Running Resettable1/1 -> Add1/2
  Demux/2 -> Abs1/1
  Demux/3 -> Abs2/1
  Compare To Constant2/1 -> Add2/1
  MinMax Running Resettable/1 -> Add1/1
  Demux/1 -> Abs/1
  Pulse Generator/1 -> MinMax Running Resettable1/2, MinMax Running Resettable/2
  Abs/1 -> Add/1
  Abs1/1 -> Add/2
  Accel/1 -> Demux/1
  MSR/1 -> Multiport Switch/4
  const/1 -> Product/1
  Divide/1 -> Compare To Constant/1, Compare To Constant2/1, Compare To Constant1/1
  Add1/1 -> Divide/1
  Multiport Switch1/1 -> Divide/2
  THRESHOLD/1 -> Multiport Switch1/2, Multiport Switch1/1
  Constant/1 -> Multiport Switch1/4
  Constant1/1 -> Multiport Switch1/3
  Constant2/1 -> Multiport Switch1/5
  Constant3/1 -> Multiport Switch1/6
  Constant4/1 -> Multiport Switch1/7
  Constant5/1 -> Multiport Switch1/8

== system Combined/Pacing/DOO/BPM to msec//B  ==
  In1 : Inport
  1 min(msec) : Constant  Value=60000  OutDataTypeStr=double
  "BPM to msec/B " : Product  Inputs=*/  OutDataTypeStr=uint16  RndMeth=Nearest
  Out1 : Outport  OutDataTypeStr=uint16
  wires:
  1 min(msec)/1 -> "BPM to msec/B "/1
  "BPM to msec/B "/1 -> Out1/1
  In1/1 -> "BPM to msec/B "/2

== system Combined/Pacing/DOOR/BPM to msec//B  ==
  OUTPUT_PACE : Inport
  1 min(msec) : Constant  Value=60000  OutDataTypeStr=double
  "BPM to msec/B " : Product  Inputs=*/  OutDataTypeStr=uint16  RndMeth=Nearest
  Out1 : Outport  OutDataTypeStr=uint16
  wires:
  1 min(msec)/1 -> "BPM to msec/B "/1
  "BPM to msec/B "/1 -> Out1/1
  OUTPUT_PACE/1 -> "BPM to msec/B "/2

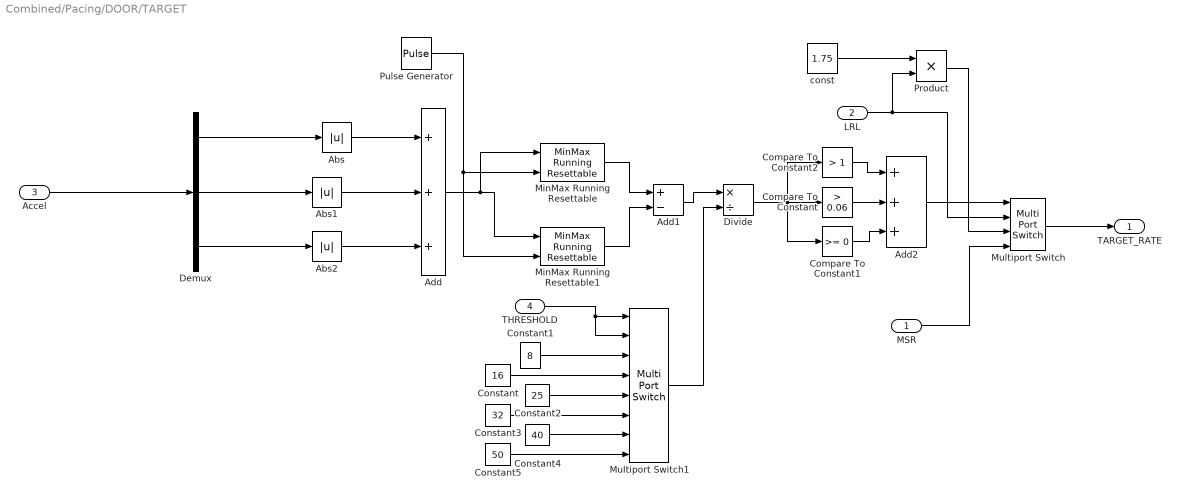
== system Combined/Pacing/DOOR/TARGET ==
  MSR : Inport
  LRL : Inport  Port=2
  Accel : Inport  Port=3
  THRESHOLD : Inport  Port=4
  Abs : Abs
  Abs1 : Abs
  Abs2 : Abs
  Add : Sum  Inputs=+++
  Add1 : Sum  Inputs=+-
  Add2 : Sum  Inputs=+++
  Compare To Constant : simulink/Logic and Bit Operations/Compare To Constant  relop=>  const=0.06  OutDataTypeStr=uint8
  Compare To Constant1 : simulink/Logic and Bit Operations/Compare To Constant  relop=>=  const=0  OutDataTypeStr=uint8
  Compare To Constant2 : simulink/Logic and Bit Operations/Compare To Constant  relop=>  const=1  OutDataTypeStr=uint8
  Constant : Constant  Value=16  OutDataTypeStr=single
  Constant1 : Constant  Value=8  OutDataTypeStr=single
  Constant2 : Constant  Value=25  OutDataTypeStr=single
  Constant3 : Constant  Value=32  OutDataTypeStr=single
  Constant4 : Constant  Value=40  OutDataTypeStr=single
  Constant5 : Constant  Value=50  OutDataTypeStr=single
  Demux : Demux  Outputs=3
  Divide : Product  Inputs=*/
  MinMax Running Resettable : simulink/Math Operations/MinMax Running Resettable  Function=max  vinit=1
  MinMax Running Resettable1 : simulink/Math Operations/MinMax Running Resettable  Function=min  vinit=1
  Multiport Switch : MultiPortSwitch  OutDataTypeStr=double
  Multiport Switch1 : MultiPortSwitch  Inputs=7
  Product : Product
  Pulse Generator : DiscretePulseGenerator  PulseType=Time based  PulseWidth=2.5
  const : Constant  Value=1.75
  TARGET_RATE : Outport
  wires:
  Compare To Constant/1 -> Add2/2
  Multiport Switch/1 -> TARGET_RATE/1
  Compare To Constant1/1 -> Add2/3
  Add2/1 -> Multiport Switch/1
  LRL/1 -> Product/2, Multiport Switch/2
  Product/1 -> Multiport Switch/3
  Abs2/1 -> Add/3
  Add/1 -> MinMax Running Resettable1/1, MinMax Running Resettable/1
  MinMax Running Resettable1/1 -> Add1/2
  Demux/2 -> Abs1/1
  Demux/3 -> Abs2/1
  Compare To Constant2/1 -> Add2/1
  MinMax Running Resettable/1 -> Add1/1
  Demux/1 -> Abs/1
  Pulse Generator/1 -> MinMax Running Resettable1/2, MinMax Running Resettable/2
  Abs/1 -> Add/1
  Abs1/1 -> Add/2
  Accel/1 -> Demux/1
  MSR/1 -> Multiport Switch/4
  const/1 -> Product/1
  Divide/1 -> Compare To Constant/1, Compare To Constant2/1, Compare To Constant1/1
  Add1/1 -> Divide/1
  Constant5/1 -> Multiport Switch1/8
  Constant3/1 -> Multiport Switch1/6
  Constant1/1 -> Multiport Switch1/3
  Constant2/1 -> Multiport Switch1/5
  Constant4/1 -> Multiport Switch1/7
  Constant/1 -> Multiport Switch1/4
  THRESHOLD/1 -> Multiport Switch1/2, Multiport Switch1/1
  Multiport Switch1/1 -> Divide/2

== system Combined/Pacing/VOO/BPM to msec//B  ==
  LRL : Inport
  1 min(msec) : Constant  Value=60000  OutDataTypeStr=double
  "BPM to msec/B " : Product  Inputs=*/  OutDataTypeStr=uint16  RndMeth=Nearest
  Out1 : Outport
  wires:
  1 min(msec)/1 -> "BPM to msec/B "/1
  "BPM to msec/B "/1 -> Out1/1
  LRL/1 -> "BPM to msec/B "/2

== system Combined/Pacing/VOOR/BPM to msec//B  ==
  OUTPUT_PACE : Inport
  1 min(msec) : Constant  Value=60000  OutDataTypeStr=double
  "BPM to msec/B " : Product  Inputs=*/  OutDataTypeStr=uint16  RndMeth=Nearest
  Out1 : Outport
  wires:
  1 min(msec)/1 -> "BPM to msec/B "/1
  "BPM to msec/B "/1 -> Out1/1
  OUTPUT_PACE/1 -> "BPM to msec/B "/2

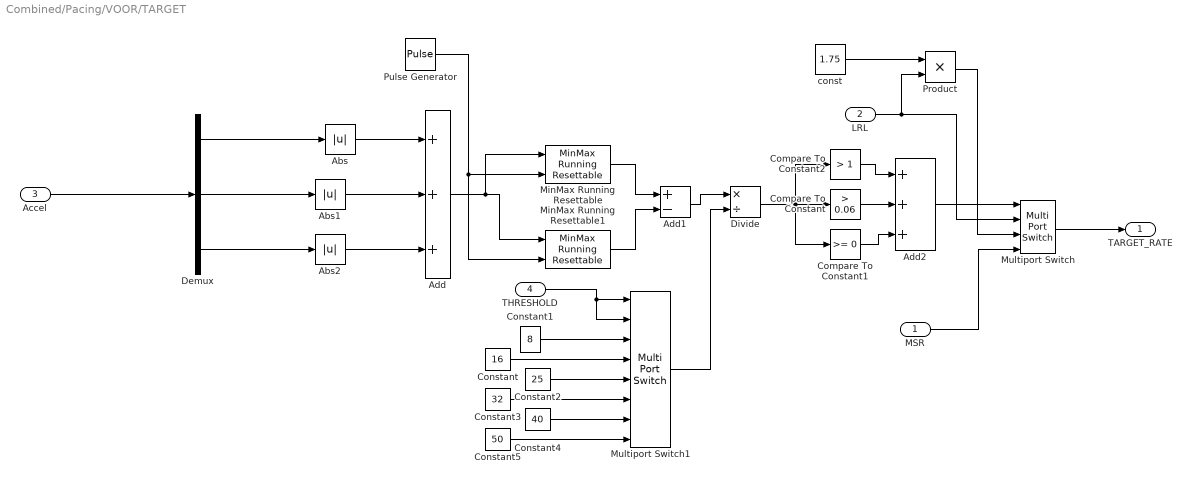
== system Combined/Pacing/VOOR/TARGET ==
  MSR : Inport
  LRL : Inport  Port=2
  Accel : Inport  Port=3
  THRESHOLD : Inport  Port=4
  Abs : Abs
  Abs1 : Abs
  Abs2 : Abs
  Add : Sum  Inputs=+++
  Add1 : Sum  Inputs=+-
  Add2 : Sum  Inputs=+++
  Compare To Constant : simulink/Logic and Bit Operations/Compare To Constant  relop=>  const=0.06  OutDataTypeStr=uint8
  Compare To Constant1 : simulink/Logic and Bit Operations/Compare To Constant  relop=>=  const=0  OutDataTypeStr=uint8
  Compare To Constant2 : simulink/Logic and Bit Operations/Compare To Constant  relop=>  const=1  OutDataTypeStr=uint8
  Constant : Constant  Value=16  OutDataTypeStr=single
  Constant1 : Constant  Value=8  OutDataTypeStr=single
  Constant2 : Constant  Value=25  OutDataTypeStr=single
  Constant3 : Constant  Value=32  OutDataTypeStr=single
  Constant4 : Constant  Value=40  OutDataTypeStr=single
  Constant5 : Constant  Value=50  OutDataTypeStr=single
  Demux : Demux  Outputs=3
  Divide : Product  Inputs=*/
  MinMax Running Resettable : simulink/Math Operations/MinMax Running Resettable  Function=max  vinit=1
  MinMax Running Resettable1 : simulink/Math Operations/MinMax Running Resettable  Function=min  vinit=1
  Multiport Switch : MultiPortSwitch  OutDataTypeStr=double
  Multiport Switch1 : MultiPortSwitch  Inputs=7
  Product : Product
  Pulse Generator : DiscretePulseGenerator  PulseType=Time based  PulseWidth=2.5
  const : Constant  Value=1.75
  TARGET_RATE : Outport
  wires:
  Compare To Constant/1 -> Add2/2
  Multiport Switch/1 -> TARGET_RATE/1
  Compare To Constant1/1 -> Add2/3
  Add2/1 -> Multiport Switch/1
  LRL/1 -> Product/2, Multiport Switch/2
  Product/1 -> Multiport Switch/3
  Abs2/1 -> Add/3
  Add/1 -> MinMax Running Resettable1/1, MinMax Running Resettable/1
  MinMax Running Resettable1/1 -> Add1/2
  Demux/2 -> Abs1/1
  Demux/3 -> Abs2/1
  Compare To Constant2/1 -> Add2/1
  MinMax Running Resettable/1 -> Add1/1
  Demux/1 -> Abs/1
  Pulse Generator/1 -> MinMax Running Resettable1/2, MinMax Running Resettable/2
  Abs/1 -> Add/1
  Abs1/1 -> Add/2
  Accel/1 -> Demux/1
  MSR/1 -> Multiport Switch/4
  const/1 -> Product/1
  Divide/1 -> Compare To Constant/1, Compare To Constant2/1, Compare To Constant1/1
  Add1/1 -> Divide/1
  Multiport Switch1/1 -> Divide/2
  Constant5/1 -> Multiport Switch1/8
  Constant3/1 -> Multiport Switch1/6
  Constant1/1 -> Multiport Switch1/3
  Constant2/1 -> Multiport Switch1/5
  Constant4/1 -> Multiport Switch1/7
  Constant/1 -> Multiport Switch1/4
  THRESHOLD/1 -> Multiport Switch1/2, Multiport Switch1/1

== system Combined/Pacing/VVI/BPM to msec//B  ==
  LRL : Inport
  1 min(msec) : Constant  Value=60000  OutDataTypeStr=double
  "BPM to msec/B " : Product  Inputs=*/  OutDataTypeStr=uint16  RndMeth=Nearest
  Out1 : Outport
  wires:
  1 min(msec)/1 -> "BPM to msec/B "/1
  "BPM to msec/B "/1 -> Out1/1
  LRL/1 -> "BPM to msec/B "/2

== system Combined/Pacing/VVIR/BPM to msec//B  ==
  LRL : Inport
  1 min(msec) : Constant  Value=60000  OutDataTypeStr=double
  "BPM to msec/B " : Product  Inputs=*/  OutDataTypeStr=uint16  RndMeth=Nearest
  Out1 : Outport
  wires:
  1 min(msec)/1 -> "BPM to msec/B "/1
  "BPM to msec/B "/1 -> Out1/1
  LRL/1 -> "BPM to msec/B "/2

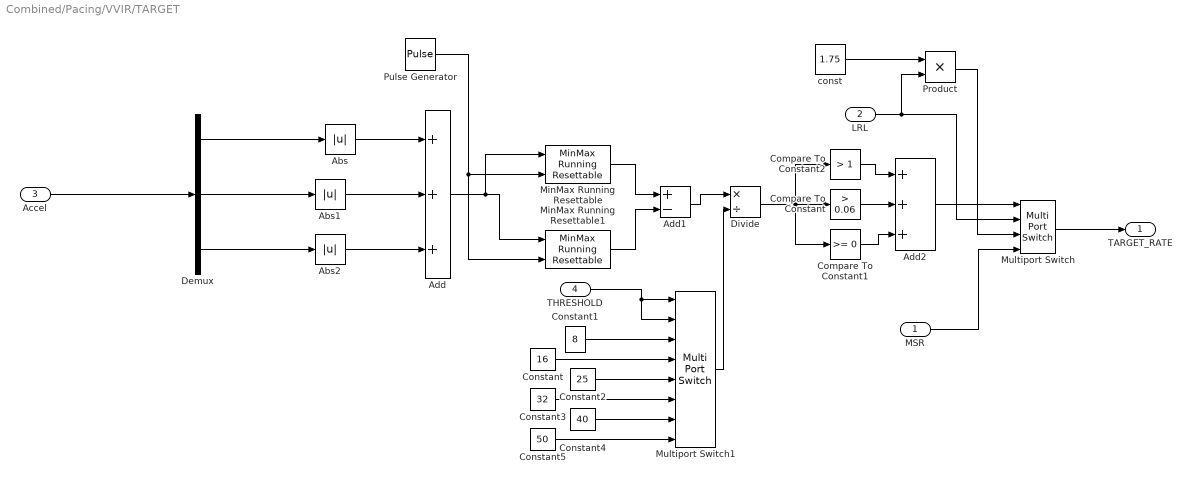
== system Combined/Pacing/VVIR/TARGET ==
  MSR : Inport
  LRL : Inport  Port=2
  Accel : Inport  Port=3
  THRESHOLD : Inport  Port=4
  Abs : Abs
  Abs1 : Abs
  Abs2 : Abs
  Add : Sum  Inputs=+++
  Add1 : Sum  Inputs=+-
  Add2 : Sum  Inputs=+++
  Compare To Constant : simulink/Logic and Bit Operations/Compare To Constant  relop=>  const=0.06  OutDataTypeStr=uint8
  Compare To Constant1 : simulink/Logic and Bit Operations/Compare To Constant  relop=>=  const=0  OutDataTypeStr=uint8
  Compare To Constant2 : simulink/Logic and Bit Operations/Compare To Constant  relop=>  const=1  OutDataTypeStr=uint8
  Constant : Constant  Value=16  OutDataTypeStr=single
  Constant1 : Constant  Value=8  OutDataTypeStr=single
  Constant2 : Constant  Value=25  OutDataTypeStr=single
  Constant3 : Constant  Value=32  OutDataTypeStr=single
  Constant4 : Constant  Value=40  OutDataTypeStr=single
  Constant5 : Constant  Value=50  OutDataTypeStr=single
  Demux : Demux  Outputs=3
  Divide : Product  Inputs=*/
  MinMax Running Resettable : simulink/Math Operations/MinMax Running Resettable  Function=max  vinit=1
  MinMax Running Resettable1 : simulink/Math Operations/MinMax Running Resettable  Function=min  vinit=1
  Multiport Switch : MultiPortSwitch  OutDataTypeStr=double
  Multiport Switch1 : MultiPortSwitch  Inputs=7
  Product : Product
  Pulse Generator : DiscretePulseGenerator  PulseType=Time based  PulseWidth=2.5
  const : Constant  Value=1.75
  TARGET_RATE : Outport
  wires:
  Compare To Constant/1 -> Add2/2
  Multiport Switch/1 -> TARGET_RATE/1
  Compare To Constant1/1 -> Add2/3
  Add2/1 -> Multiport Switch/1
  LRL/1 -> Product/2, Multiport Switch/2
  Product/1 -> Multiport Switch/3
  Abs2/1 -> Add/3
  Add/1 -> MinMax Running Resettable1/1, MinMax Running Resettable/1
  MinMax Running Resettable1/1 -> Add1/2
  Demux/2 -> Abs1/1
  Demux/3 -> Abs2/1
  Compare To Constant2/1 -> Add2/1
  MinMax Running Resettable/1 -> Add1/1
  Demux/1 -> Abs/1
  Pulse Generator/1 -> MinMax Running Resettable1/2, MinMax Running Resettable/2
  Abs/1 -> Add/1
  Abs1/1 -> Add/2
  Accel/1 -> Demux/1
  MSR/1 -> Multiport Switch/4
  const/1 -> Product/1
  Divide/1 -> Compare To Constant/1, Compare To Constant2/1, Compare To Constant1/1
  Add1/1 -> Divide/1
  Constant5/1 -> Multiport Switch1/8
  Constant3/1 -> Multiport Switch1/6
  Constant1/1 -> Multiport Switch1/3
  Constant2/1 -> Multiport Switch1/5
  Constant4/1 -> Multiport Switch1/7
  Constant/1 -> Multiport Switch1/4
  THRESHOLD/1 -> Multiport Switch1/2, Multiport Switch1/1
  Multiport Switch1/1 -> Divide/2

== stateflow chart Combined/Pacing/VOO/Chart ==
  state Charging_and_Discharging
    entry:
    PACE_GND_CTRL=true;
    ATR_PACE_CTRL=false;
    VENT_PACE_CTRL=false;
    PACING_REF_PWM=uint8(Amplitude*20);
    PACE_CHARGE_CTRL=true;
    Z_ATR_CTRL=false;
    Z_VENT_CTRL=false;
    ATR_GND_CTRL=false;
    VENT_GND_CTRL=true;
  state V_Pacing
    entry:
    PACE_CHARGE_CTRL=false;
    PACE_GND_CTRL=true;
    ATR_GND_CTRL=false;
    Z_ATR_CTRL=false;
    Z_VENT_CTRL=false;
    VENT_GND_CTRL=false;
    ATR_PACE_CTRL=false;
    VENT_PACE_CTRL=true;
  (default) -> Charging_and_Discharging
  Charging_and_Discharging -> V_Pacing : after(LRL-PULSE_WIDTH, msec)
  V_Pacing -> Charging_and_Discharging : after(PULSE_WIDTH, msec)
  data: ATR_PACE_CTRL output boolean; VENT_PACE_CTRL output boolean; PACING_REF_PWM output uint8; Amplitude input double; PACE_CHARGE_CTRL output boolean; ATR_GND_CTRL output boolean; Z_ATR_CTRL output boolean; Z_VENT_CTRL output boolean; VENT_GND_CTRL output boolean; PACE_GND_CTRL output boolean; PULSE_WIDTH input uint16; LRL input uint16

== stateflow chart Combined/Pacing ==
  state INIT
  state AOO
  state VOO
  state AAI
  state VVI
  state DOO
  state AOOR
  state VOOR
  state AAIR
  state VVIR
  state DOOR
  (default) -> INIT
  AOO -> INIT : [MODE~=1]
  INIT -> AOO [order 5] : [MODE==1]
  VOO -> INIT : [MODE~=2]
  INIT -> VOO [order 6] : [MODE==2]
  AAI -> INIT : [MODE~=3]
  INIT -> AAI [order 2] : [MODE==3]
  VVI -> INIT : [MODE~=4]
  INIT -> VVI [order 3] : [MODE==4]
  DOO -> INIT : [MODE~=5]
  INIT -> DOO [order 7] : [MODE==5]
  AOOR -> INIT : [MODE~=6]
  INIT -> AOOR [order 8] : [MODE==6]
  VOOR -> INIT : [MODE~=7]
  INIT -> VOOR [order 1] : [MODE==7]
  AAIR -> INIT : [MODE~=8]
  INIT -> AAIR [order 9] : [MODE==8]
  VVIR -> INIT : [MODE~=9]
  INIT -> VVIR [order 10] : [MODE==9]
  DOOR -> INIT : [MODE~=10]
  INIT -> DOOR [order 4] : [MODE==10]
  data: sf_internal_action_state_placeholder_data local double size=1 =0; sf_internal_action_state_placeholder_data local double size=1 =0; sf_internal_action_state_placeholder_data local double size=1 =0; sf_internal_action_state_placeholder_data local double size=1 =0; sf_internal_action_state_placeholder_data local double size=1 =0; sf_internal_action_state_placeholder_data local double size=1 =0; sf_internal_action_state_placeholder_data local double size=1 =0; sf_internal_action_state_placeholder_data local double size=1 =0; sf_internal_action_state_placeholder_data local double size=1 =0; sf_internal_action_state_placeholder_data local double size=1 =0; ATR_CMP_DETECT input; VENT_CMP_DETECT input; Accel input; MODE input uint8; ATR_AMP input double; Pulse_Width_atrium input uint16; LRL input uint16; ATR_PACE_CTRL output boolean; VENT_PACE_CTRL output boolean; PACING_REF_PWM output uint8; PACE_CHARGE_CTRL output boolean; ATR_GND_CTRL output boolean; Z_ATR_CTRL output boolean; Z_VENT_CTRL output boolean; VENT_GND_CTRL output boolean; PACE_GND_CTRL output boolean; APR input uint16; VRP input int16; Pulse_Width_ventricle input uint16; AV_DEALAY input uint16; reaction input; recovery input; threshold input; MSR input; VENT_AMP input double
